simulink model "fwr"  (R2021a)
settings: Solver=VariableStepAuto  StartTime=0.0  StopTime=0.06  RelTol=1e-3
libraries: spsDiodeLib x8, spsSeriesRLCBranchLib x3, spsVoltageMeasurementLib x3, spsACVoltageSourceLib x2, spsGroundLib x2, spsLinearTransformerLib x2, spspowerguiLib x1
settings Model: Creator=SREETAM  LastModifiedBy=SREETAM

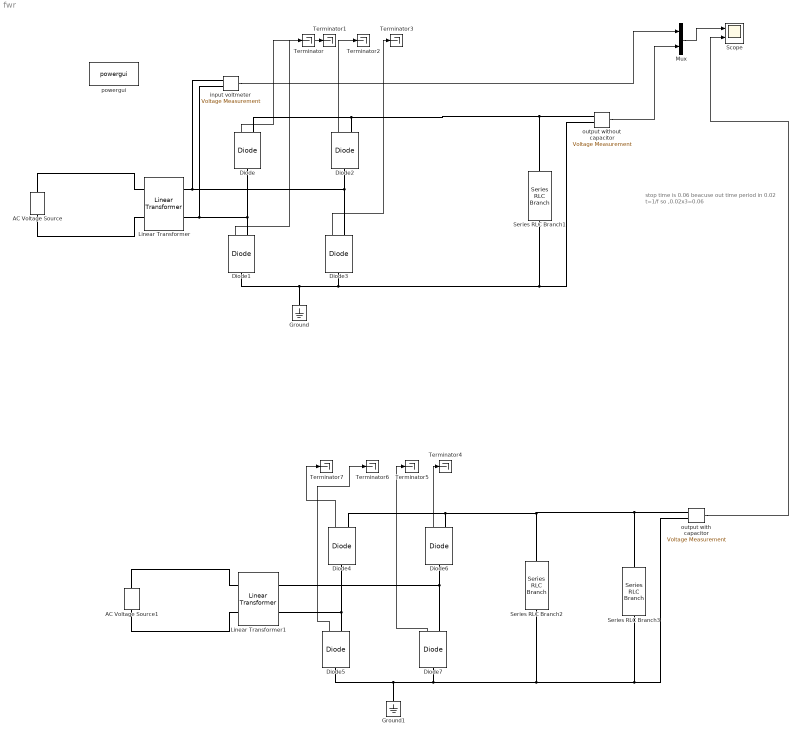
== system fwr ==
  note: stop time is 0.06 beacuse out time period in 0.02
      | t=1/f
      | so ,0.02x3=0.06
  AC Voltage Source : spsACVoltageSourceLib/AC Voltage Source  Amplitude=220  Phase=0  Frequency=50  SampleTime=0  Measurements=None  BusType=swing  Pref=10e3  Qref=0  Qmin=-inf  Qmax=+inf
  AC Voltage Source1 : spsACVoltageSourceLib/AC Voltage Source  Amplitude=220  Phase=0  Frequency=50  SampleTime=0  Measurements=None  BusType=swing  Pref=10e3  Qref=0  Qmin=-inf  Qmax=+inf
  Diode{,1..7} (8 alike) : spsDiodeLib/Diode  Ron=0.001  Lon=0  Vf=0.8  IC=0  UseSnubber=0  Rs=500  Cs=250e-9  Measurements=on
  Ground : spsGroundLib/Ground  LConnTagsString=a
  Ground1 : spsGroundLib/Ground  LConnTagsString=a
  Linear Transformer : spsLinearTransformerLib/Linear Transformer  UNITS=SI  NominalPower=[ 1e3 50 ]  winding1=[2 0 0]  winding2=[1 0 0]  ThreeWindings=off  winding3=[3.15e+05 0.7938 0.084225]  RmLm=[inf inf ]  Measurements=None  DataType=on
  Linear Transformer1 : spsLinearTransformerLib/Linear Transformer  UNITS=SI  NominalPower=[ 1e3 50 ]  winding1=[2 0 0]  winding2=[1 0 0]  ThreeWindings=off  winding3=[3.15e+05 0.7938 0.084225]  RmLm=[inf inf ]  Measurements=None  DataType=on
  Mux : Mux  Inputs=2
  Scope : Scope  NumInputPorts=2
  Series RLC Branch1 : spsSeriesRLCBranchLib/Series RLC Branch  LConnTagsString=__new0  RConnTagsString=__new0  BranchType=R  Resistance=1000  Inductance=1e-3  SetiL0=off  InitialCurrent=0  Capacitance=1e-6  Setx0=off  InitialVoltage=0  Measurements=None
  Series RLC Branch2 : spsSeriesRLCBranchLib/Series RLC Branch  LConnTagsString=__new0  RConnTagsString=__new0  BranchType=R  Resistance=1000  Inductance=1e-3  SetiL0=off  InitialCurrent=0  Capacitance=1e-6  Setx0=off  InitialVoltage=0  Measurements=None
  Series RLC Branch3 : spsSeriesRLCBranchLib/Series RLC Branch  LConnTagsString=__new0  RConnTagsString=__new0  BranchType=C  Resistance=0  Inductance=1e-3  SetiL0=off  InitialCurrent=0  Capacitance=0.35  Setx0=off  InitialVoltage=0  Measurements=None
  Terminator{,1..7} (8 alike) : Terminator
  input voltmeter : spsVoltageMeasurementLib/Voltage Measurement  PhasorSimulation=off  OutputType=Complex  PSBequivalent=0
  output with capacitor : spsVoltageMeasurementLib/Voltage Measurement  PhasorSimulation=off  OutputType=Complex  PSBequivalent=0
  output without capacitor : spsVoltageMeasurementLib/Voltage Measurement  PhasorSimulation=off  OutputType=Complex  PSBequivalent=0
  powergui : spspowerguiLib/powergui  Priority=1  SimulationMode=Continuous  SampleTime=50e-6  frequency=60  Iterations=50  frequencyindice=50  Pbase=100e6  ErrMax=1e-4  UnitsV=kV  UnitsW=MW  buscounter=0  FunctionMessages=off  echomessages=off  EnableUseOfTLC=off  CurrentSourceSwitches=off  DisableSnubberDevices=off  DisableRonSwitches=off  DisableVfSwitches=off  DisplayEquations=off  AutomaticDiscreteSolvers=off  SolverType=Tustin/Backward Euler (TBE)  Interpol=off  ExternalGateDelay=off  methode=off  Ts=100  x0status=blocks  SPID=on  SwTol=0  HookPort=off  NonlinearTolerance=1e-4  nMaxIteration=100  ContinueOnMaxIteration=off  RestoreLinks=warning  ResistiveCurrentMeasurement=off  Frange=[0:2:500]  Ylog=off  Xlog=on  ShowGrid=off  save=off  variable=ZData  structure=0  ZoomFFT=off  StartTime=0.0  cycles=1  DisplayStyle=1  fundamental=60  FreqAxis=off  MaxFrequency=1000  frequencyindicesteady=1  RmsSteady=1  display=off
  wires:
  input voltmeter/1 -> Mux/1
  output without capacitor/1 -> Mux/2
  Mux/1 -> Scope/1
  output with capacitor/1 -> Scope/2
  Diode/1 -> Terminator/1
  Diode2/1 -> Terminator2/1
  Diode4/1 -> Terminator7/1
  Diode5/1 -> Terminator6/1
  Diode7/1 -> Terminator5/1
  Diode6/1 -> Terminator4/1
  Diode1/1 -> Terminator1/1
  Diode3/1 -> Terminator3/1
  connections:
  AC Voltage Source/LConn1 -- Linear Transformer/LConn2
  AC Voltage Source/RConn1 -- Linear Transformer/LConn1
  Diode3/RConn1 -- input voltmeter/LConn1 -- Linear Transformer/RConn1 -- Diode2/LConn1
  Diode1/RConn1 -- input voltmeter/LConn2 -- Linear Transformer/RConn2 -- Diode/LConn1
  Diode1/LConn1 -- Ground/LConn1 -- Series RLC Branch1/RConn1 -- output without capacitor/LConn2 -- Diode3/LConn1
  Diode/RConn1 -- Series RLC Branch1/LConn1 -- output without capacitor/LConn1 -- Diode2/RConn1
  Diode7/LConn1 -- Series RLC Branch3/RConn1 -- output with capacitor/LConn2 -- Series RLC Branch2/RConn1 -- Diode5/LConn1 -- Ground1/LConn1
  Diode4/LConn1 -- Linear Transformer1/RConn2 -- Diode5/RConn1
  Diode6/RConn1 -- Diode4/RConn1 -- Series RLC Branch3/LConn1 -- output with capacitor/LConn1 -- Series RLC Branch2/LConn1
  Linear Transformer1/RConn1 -- Diode7/RConn1 -- Diode6/LConn1
  AC Voltage Source1/LConn1 -- Linear Transformer1/LConn2
  AC Voltage Source1/RConn1 -- Linear Transformer1/LConn1
